simulink subsystem "translation_model"  (R2025b)
settings: Solver=VariableStepAuto  StartTime=0.0  StopTime=10.0  RelTol=1e-3
values from neighbouring files (symbols this model uses):
  g = 9.81    [params.m]    (also in params_1dof.m; params_3dof.m)
  m = 1.014    [params.m]    (also in params_1dof.m; params_3dof.m)
settings Model: Creator=schwmaxi  LastModifiedBy=schwmaxi

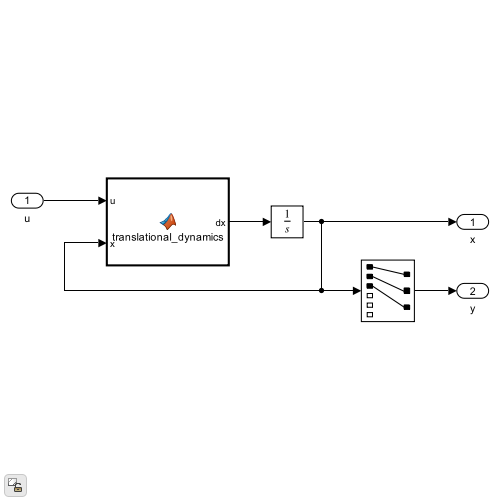
[thumbnail: Simulink's stored preview of the top-level diagram]
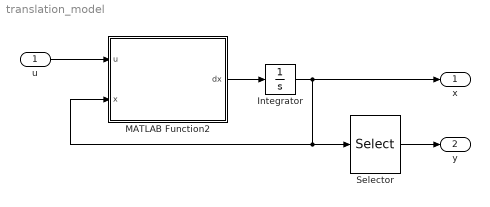
== system translation_model ==
  u : Inport
  Integrator : Integrator  InitialCondition=[0; 0; 0; 0; 0; 0]
  MATLAB Function2 : MATLAB Function  TreatAsAtomicUnit=on
  Selector : Selector  InputPortWidth=6  IndexOptions=Index vector (dialog)  Indices=[1 2 3]  OutputSizes=1
  x : Outport
  y : Outport  Port=2
  wires:
  MATLAB Function2/1(dx) -> Integrator/1
  u/1 -> MATLAB Function2/1(u)
  Selector/1 -> y/1
  Integrator/1 -> Selector/1, MATLAB Function2/2(x), x/1

== matlab function translation_model/MATLAB Function2 ==
  data: u input; x input; dx output; m parameter; g parameter
function dx = translational_dynamics(u, x, m, g)
    % m und g werden als Parameter Data übergeben, vgl. Symbols Pane
    thrust = u(1);
    euler_angles = u(2:4);

    phi = euler_angles(1);
    theta = euler_angles(2);
    psi = euler_angles(3);

    % Elementarmatrizen
    R_x = [1, 0, 0; 
           0, cos(phi), -sin(phi); 
           0, sin(phi), cos(phi)];
    
    R_y = [cos(theta), 0, sin(theta); 
           0, 1, 0; 
           -sin(theta), 0, cos(theta)];
    
    R_z = [cos(psi), -sin(psi), 0; 
           sin(psi), cos(psi), 0; 
           0, 0, 1];

    % Gesamt-Rotationsmatrix (Body to World: R = Rz * Ry * Rx)
    R = R_z * R_y * R_x;

    position_dot = x(4:6);
    velocity_dot = [0; 0; -g] +1/m * R * [0; 0; thrust];

    dx = [position_dot; velocity_dot];
end
